simulink model "Control_Logic_e"  (R2019b)
settings: Solver=FixedStepAuto  StartTime=0  StopTime=200  FixedStep=0.1  RelTol=1e-3
values from neighbouring files (symbols this model uses):
  Sample_time = 1    [test_tool_ini.m]    (also in test_tool_initialize.m = 0.1)
undefined symbols (not defined in the file or in its folder): Aset_N1, Aset_N10, Aset_N11, Aset_N12, Aset_N2, Aset_N3, Aset_N4, Aset_N5, Aset_N6, Aset_N7, Aset_N8, Aset_N9, Dset_N1, Dset_N2
(part 1 of 3)
settings Model: Creator=M156732  LastModifiedBy=yangy
settings DataIOCC: ExternalInput=aoe_tsinghua_mhi_data  LoadExternalInput=on  ReturnWorkspaceOutputs=off
settings DebuggingCC: UnderSpecifiedDimensionMsg=warning  ArithmeticOperatorsInVariantConditions=warning
settings ModelReferenceCC: ModelReferenceNumInstancesAllowed=Single
settings SFSimCC: CustomCodeUndefinedFunction=UseInterfaceOnly

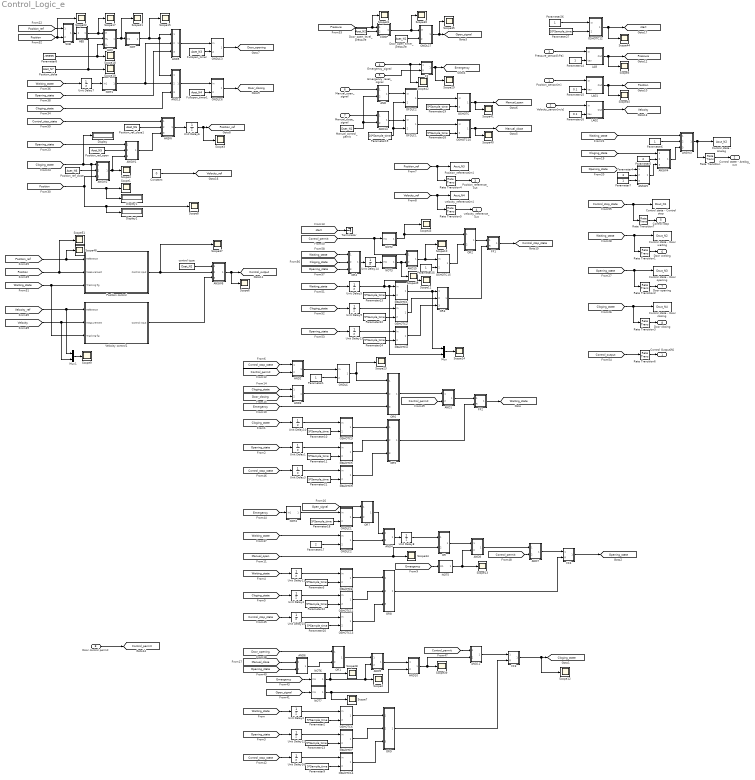
== system Control_Logic_e ==
  Position_sensor[m] : Inport  OutDataTypeStr=double  Unit=mm  PortDimensions=1  SampleTime=Sample_time
  Velocity_sensor[m/s] : Inport  Port=2  OutDataTypeStr=double  Unit=mm  PortDimensions=1  SampleTime=Sample_time
  Pressure_sensor[kPa] : Inport  Port=3  OutDataTypeStr=double  Unit=kPa  PortDimensions=1  SampleTime=Sample_time
  Emergency_signal : Inport  Port=4  OutDataTypeStr=boolean  PortDimensions=1  SampleTime=Sample_time
  Emergency_reset_signal : Inport  Port=5  OutDataTypeStr=boolean  PortDimensions=1  SampleTime=Sample_time
  Manual_open_signal : Inport  Port=6  OutDataTypeStr=boolean  PortDimensions=1  SampleTime=Sample_time
  Manual_close_signal : Inport  Port=7  OutDataTypeStr=boolean  PortDimensions=1  SampleTime=Sample_time
  Door control permit : Inport  Port=8  OutDataTypeStr=boolean  PortDimensions=1  SampleTime=Sample_time
  ABS : Subsystem
  AND : Subsystem
  AND1 : Subsystem
  AND10 : Subsystem
  AND11 : Subsystem
  AND13 : Subsystem
  AND14 : Subsystem
  AND15 : Subsystem
  AND2 : Subsystem
  AND3 : Subsystem
  AND4 : Subsystem
  AND5 : Subsystem
  AND6 : Subsystem
  AND7 : Subsystem
  AND8 : Subsystem
  AND9 : Subsystem
  ANSW : Subsystem
  ANSW1 : Subsystem
  ANSW2 : Subsystem
  ANSW3 : Subsystem
  ANSW4 : Subsystem
  ANSW5 : Subsystem
  ANSW6 : Subsystem
  COMP : Subsystem
  Constant : Constant  Value=0
  Control state - Analog : ToWorkspace  VariableName=Aout_N2  SampleTime=Sample_time
  Control state - Control stop : ToWorkspace  VariableName=Dout_N1  SampleTime=Sample_time
  Control state - Door closing : ToWorkspace  VariableName=Dout_N4  SampleTime=Sample_time
  Control state - Door opening : ToWorkspace  VariableName=Dout_N3  SampleTime=Sample_time
  Control state - Door waiting : ToWorkspace  VariableName=Dout_N2  SampleTime=Sample_time
  Display : Display
  Display1 : Display
  Display2 : Display
  Door_open_level_pressure : Constant  Value=Aset_N2  OutDataTypeStr=double  SampleTime=Sample_time
  Door_open_timer_pressure : Constant  Value=Aset_N1  OutDataTypeStr=double  SampleTime=Sample_time
  FF : Subsystem
  FF1 : Subsystem
  FF2 : Subsystem
  FF3 : Subsystem
  FF4 : Subsystem
  Fullopen_timer : Constant  Value=Aset_N3  OutDataTypeStr=double  SampleTime=Sample_time
  Fullopen_timer1 : Constant  Value=Aset_N4  OutDataTypeStr=double  SampleTime=Sample_time
  HLM : Subsystem
  LAG : Subsystem
  LAG1 : Subsystem
  LAG2 : Subsystem
  Manual_control_pemit : Constant  Value=Dset_N1  OutDataTypeStr=boolean  SampleTime=Sample_time
  Mux : Mux  Inputs=2
  Mux1 : Mux  Inputs=2
  NOT : Subsystem
  NOT1 : Subsystem
  NOT2 : Subsystem
  NOT3 : Subsystem
  NOT4 : Subsystem
  NOT5 : Subsystem
  NOT6 : Subsystem
  NOT7 : Subsystem
  OFDLC1 : Subsystem
  OFDLC2 : Subsystem
  ONDLC : Subsystem
  ONDLC1 : Subsystem
  ONDLC2 : Subsystem
  ONDLC3 : Subsystem
  ONDLC6 : Subsystem
  ONDLC7 : Subsystem
  OR : Subsystem
  OR1 : Subsystem
  OR2 : Subsystem
  OR3 : Subsystem
  OR4 : Subsystem
  OR5 : Subsystem
  OR6 : Subsystem
  OR7 : Subsystem
  OR8 : Subsystem
  OR9 : Subsystem
  OSHOTC : Subsystem
  OSHOTC1 : Subsystem
  OSHOTC10 : Subsystem
  OSHOTC11 : Subsystem
  OSHOTC12 : Subsystem
  OSHOTC13 : Subsystem
  OSHOTC14 : Subsystem
  OSHOTC15 : Subsystem
  OSHOTC2 : Subsystem
  OSHOTC3 : Subsystem
  OSHOTC4 : Subsystem
  OSHOTC5 : Subsystem
  OSHOTC6 : Subsystem
  OSHOTC7 : Subsystem
  OSHOTC8 : Subsystem
  OSHOTC9 : Subsystem
  Parameter{1,6..7,14,25} (5 alike) : Constant  OutDataTypeStr=double  SampleTime=Sample_time
  Parameter{2..3,9..13,18,20..24,28..29} (15 alike) : Constant  Value=5*Sample_time  OutDataTypeStr=double  SampleTime=Sample_time
  Parameter15 : Constant  Value=0.1  OutDataTypeStr=double  SampleTime=Sample_time
  Parameter16 : Constant  Value=0.1  OutDataTypeStr=double  SampleTime=Sample_time
  Parameter17 : Constant  Value=2  OutDataTypeStr=double  SampleTime=Sample_time
  Parameter19 : Constant  Value=10*Sample_time  OutDataTypeStr=double  SampleTime=Sample_time
  Parameter26 : Constant  OutDataTypeStr=boolean  SampleTime=Sample_time
  Parameter27 : Constant  Value=10*Sample_time  OutDataTypeStr=double  SampleTime=Sample_time
  Parameter4 : Constant  Value=3  OutDataTypeStr=double  SampleTime=Sample_time
  Parameter5 : Constant  Value=2  OutDataTypeStr=double  SampleTime=Sample_time
  Parameter8 : Constant  Value=-99999  OutDataTypeStr=double  SampleTime=Sample_time
  Position control : Subsystem
  Position_delta : Constant  Value=Aset_N7  OutDataTypeStr=double  SampleTime=Sample_time
  Position_ref_close : Constant  Value=Aset_N6  OutDataTypeStr=double  SampleTime=Sample_time
  Position_ref_close1 : Constant  Value=Aset_N6  OutDataTypeStr=double  SampleTime=Sample_time
  Position_ref_open : Constant  Value=Aset_N5  OutDataTypeStr=double  SampleTime=Sample_time
  Position_reference[m] : ToWorkspace  VariableName=Aout_N3  SampleTime=Sample_time
  Rate Transition{,1..7} (8 alike) : RateTransition  OutPortSampleTime=Sample_time
  SUB : Subsystem
  Scope{1..15,17..19,21..23,28..31,34..35,37,39..45,48..49,51} (38 alike) : Scope
  Terminator : Terminator
  Unit Delay{1..13,15..16} (15 alike) : UnitDelay  SampleTime=Sample_time  HasFrameUpgradeWarning=on
  Unit Delay14 : UnitDelay  InitialCondition=1  SampleTime=Sample_time  HasFrameUpgradeWarning=on
  Velocity control1 : Subsystem
  control type : Constant  Value=Dset_N2  OutDataTypeStr=boolean  SampleTime=Sample_time
  velocity_reference[m] : ToWorkspace  VariableName=Aout_N4  SampleTime=Sample_time
  Control Output[N] : Outport  OutDataTypeStr=double  Unit=N  SampleTime=Sample_time  VectorParamsAs1DForOutWhenUnconnected=off  LockScale=on
  Control state - Analog_out : Outport  Port=2  SampleTime=Sample_time  VectorParamsAs1DForOutWhenUnconnected=off
  Position_reference_out : Outport  Port=3  SampleTime=Sample_time  VectorParamsAs1DForOutWhenUnconnected=off
  velocity_reference_out : Outport  Port=4  SampleTime=Sample_time  VectorParamsAs1DForOutWhenUnconnected=off
  Control stop : Outport  Port=5  SampleTime=Sample_time  VectorParamsAs1DForOutWhenUnconnected=off
  Door waiting : Outport  Port=6  SampleTime=Sample_time  VectorParamsAs1DForOutWhenUnconnected=off
  Door opening : Outport  Port=7  SampleTime=Sample_time  VectorParamsAs1DForOutWhenUnconnected=off
  Door closing : Outport  Port=8  SampleTime=Sample_time  VectorParamsAs1DForOutWhenUnconnected=off
  tag scope: Cloging_state=global, Control_output=global, Control_permit=global, Control_stop_state=global, Door_closing=global, Door_opening=global, Emergency=global, Manual_close=global, Manual_open=global, Open_signal=global, Opening_state=global, Position=global, Position_ref=global, Pressure=global, Velocity=global, Velocity_ref=global, Waiting_state=global, start=global
  wires:
  FF3/1(Out1) -> [Cloging_state], Scope12/1
  FF4/1(Out1) -> [Opening_state]
  AND3/1(Out1) -> OR6/2(In2)
  [Emergency] -> OR6/3(In3)
  [Door_closing] -> AND3/2(In2)
  [Cloging_state] -> AND3/1(In1)
  [Manual_open] -> OR/2(In2), Scope34/1
  OR/1(Out) -> AND8/1(In1)
  [Door_opening] -> OR1/1(In1)
  Door_open_timer_pressure/1 -> ONDLC7/2(Tset)
  Door_open_level_pressure/1 -> COMP/2(In2)
  COMP/1(Out1) -> ONDLC7/1(In), Scope30/1
  ONDLC7/1(Out) -> Scope35/1, [Open_signal]
  FF/1(Out1) -> Scope29/1, [Emergency]
  Emergency_reset_signal/1 -> FF/2(R)
  ANSW4/1(Out1) -> ANSW3/3(InB)
  ANSW5/1(Out1) -> ANSW4/3(InB)
  Parameter4/1 -> ANSW5/2(InA)
  Parameter5/1 -> ANSW4/2(InA)
  Parameter6/1 -> ANSW3/2(InA)
  Parameter7/1 -> ANSW5/3(InB)
  ANSW3/1(Out1) -> Rate Transition/1, Control state - Analog/1
  Manual_control_pemit/1 -> AND14/2(In2), AND/2(In2)
  [Position_ref] -> SUB/1(In1)
  SUB/1(Out) -> ABS/1(In1)
  Position_delta/1 -> HLM/2(HL), Scope19/1
  Parameter8/1 -> HLM/3(LL), Scope18/1
  HLM/1(Out1) -> NOT/1(In1), Scope21/1
  Fullopen_timer/1 -> ONDLC3/2(Tset)
  [Opening_state] -> ANSW1/1(SW)
  ANSW2/1(Out1) -> ANSW1/3(InB), Scope4/1
  [Cloging_state] -> Display/1, Display1/1, Scope1/1, ANSW2/1(SW)
  Position_ref_open/1 -> ANSW1/2(InA)
  Position_ref_close/1 -> ANSW2/2(InA)
  [Position] -> ANSW2/3(InB), Display2/1, Scope8/1
  Fullopen_timer1/1 -> ONDLC6/2(Tset)
  [Waiting_state] -> Rate Transition1/1, Control state - Door waiting/1
  [Opening_state] -> Rate Transition2/1, Control state - Door opening/1
  [Cloging_state] -> Rate Transition3/1, Control state - Door closing/1
  [Position] -> SUB/2(In2), Scope22/1
  [Pressure] -> COMP/1(In1), Scope31/1
  AND2/1(Out1) -> ONDLC/1(In)
  ONDLC/1(Out) -> OR6/1(In1), Scope23/1
  ABS/1(Out1) -> HLM/1(In), Scope17/1
  ONDLC3/1(Out) -> [Door_opening]
  ONDLC6/1(Out) -> [Door_closing]
  [Waiting_state] -> Unit Delay7/1
  NOT/1(Out1) -> Scope15/1, AND13/1(In1), AND5/1(In1)
  AND5/1(Out1) -> ONDLC3/1(In)
  NOT1/1(Out1) -> AND5/2(In2), AND13/2(In2)
  Unit Delay7/1 -> NOT1/1(In1)
  AND4/1(Out1) -> Unit Delay8/1
  Unit Delay8/1 -> OR/1(In1)
  [Opening_state] -> AND5/3(In3)
  [Cloging_state] -> AND13/3(In3)
  AND13/1(Out1) -> ONDLC6/1(In)
  [Opening_state] -> Unit Delay1/1
  [Cloging_state] -> Unit Delay10/1
  Unit Delay10/1 -> OSHOTC3/1(In)
  Unit Delay1/1 -> OSHOTC5/1(In)
  OSHOTC5/1(Out) -> OR5/2(In2)
  OSHOTC11/1(Out) -> OR8/2(In2)
  [Waiting_state] -> Unit Delay11/1
  OSHOTC8/1(Out) -> OR8/1(In1)
  Unit Delay11/1 -> OSHOTC8/1(In)
  [Cloging_state] -> Unit Delay4/1
  Unit Delay4/1 -> OSHOTC11/1(In)
  [Waiting_state] -> Unit Delay2/1
  Parameter2/1 -> OSHOTC6/2(Tset)
  OSHOTC6/1(Out) -> OR9/1(In1)
  Parameter13/1 -> OSHOTC7/2(Tset)
  [Opening_state] -> Unit Delay12/1
  OSHOTC7/1(Out) -> OR9/2(In2)
  Unit Delay2/1 -> OSHOTC6/1(In)
  Unit Delay12/1 -> OSHOTC7/1(In)
  Pressure_sensor[kPa]/1 -> LAG/1(In)
  LAG/1(Out) -> [Pressure], Scope5/1
  LAG1/1(Out) -> Scope45/1, [Position]
  Position_sensor[m]/1 -> LAG1/1(In)
  LAG2/1(Out) -> [Velocity]
  Velocity_sensor[m/s]/1 -> LAG2/1(In)
  Parameter14/1 -> LAG/2(tau)
  Parameter15/1 -> LAG1/2(tau)
  Parameter16/1 -> LAG2/2(tau)
  [Waiting_state] -> ANSW3/1(SW)
  [Cloging_state] -> ANSW4/1(SW)
  [Opening_state] -> ANSW5/1(SW)
  Rate Transition/1 -> Control state - Analog_out/1
  Rate Transition1/1 -> Door waiting/1
  Rate Transition2/1 -> Door opening/1
  Rate Transition3/1 -> Door closing/1
  [Waiting_state] -> ONDLC2/1(In)
  ONDLC2/1(Out) -> AND4/2(In2)
  [Position_ref] -> Rate Transition4/1, Position_reference[m]/1
  Rate Transition4/1 -> Position_reference_out/1
  Rate Transition5/1 -> velocity_reference_out/1
  [Velocity_ref] -> velocity_reference[m]/1, Rate Transition5/1
  [Emergency] -> NOT5/1(In1)
  NOT5/1(Out1) -> AND8/2(In2), Scope13/1
  [Emergency] -> NOT6/1(In1)
  OR1/1(Out) -> AND9/1(In1)
  OR7/1(Out) -> AND4/1(In1)
  [Open_signal] -> OR7/1(In1)
  [Emergency] -> NOT4/1(In1)
  Parameter18/1 -> ONDLC1/2(Tset)
  ONDLC1/1(Out) -> OR7/2(In2)
  NOT4/1(Out1) -> ONDLC1/1(In)
  Manual_open_signal/1 -> AND/1(In1)
  Manual_close_signal/1 -> AND14/1(In1)
  AND14/1(Out1) -> OFDLC1/1(In)
  AND/1(Out1) -> OFDLC2/1(In)
  Parameter19/1 -> OFDLC1/2(Tset), OFDLC2/2(Tset)
  AND6/1(Out1) -> OR1/2(In2)
  [Opening_state] -> AND6/2(In2)
  [Open_signal] -> NOT7/1(In1)
  NOT7/1(Out1) -> AND10/2(In2), Scope7/1
  NOT6/1(Out1) -> Scope28/1, AND9/2(In2), Scope2/1
  Emergency_signal/1 -> FF/1(SS), Scope42/1
  AND9/1(Out1) -> AND10/1(In1)
  Door control permit/1 -> [Control_permit]
  OSHOTC13/1(Out) -> OR8/3(In3)
  OSHOTC9/1(Out) -> OR5/3(In3)
  AND11/1(Out1) -> FF3/1(SS)
  AND10/1(Out1) -> AND11/2(In2), Scope39/1
  [Control_permit] -> AND11/1(In1)
  AND8/1(Out1) -> AND7/1(In1)
  [Control_permit] -> AND7/2(In2)
  [Control_permit] -> AND1/2(In2)
  OR6/1(Out) -> AND1/1(In1)
  AND1/1(Out1) -> FF2/1(SS)
  FF1/1(Out1) -> [Control_stop_state]
  [Control_permit] -> AND15/1(In1), NOT2/1(In1)
  OSHOTC4/1(Out) -> OR3/3(In3)
  Unit Delay9/1 -> OSHOTC2/1(In)
  [Cloging_state] -> Unit Delay9/1
  Unit Delay5/1 -> Scope11/1, Mux/2, OSHOTC1/1(In)
  OSHOTC1/1(Out) -> Mux/1, OR3/1(In1)
  [Waiting_state] -> Unit Delay5/1
  OSHOTC2/1(Out) -> OR3/2(In2)
  Unit Delay13/1 -> OSHOTC4/1(In)
  [Opening_state] -> Unit Delay13/1
  OR3/1(Out) -> FF1/2(R)
  Rate Transition6/1 -> Control Output[N]/1
  [Control_output] -> Rate Transition6/1
  Rate Transition7/1 -> Control stop/1
  [Control_stop_state] -> Control state - Control stop/1, Rate Transition7/1
  Constant/1 -> [Velocity_ref]
  NOT2/1(Out1) -> OR2/1(In1), Scope43/1
  OR2/1(Out) -> FF1/1(SS)
  [Cloging_state] -> OR4/2(In2)
  Unit Delay14/1 -> NOT3/1(In1)
  [Waiting_state] -> OR4/1(In1)
  OR4/1(Out) -> Unit Delay14/1
  [Opening_state] -> OR4/3(In3)
  [Control_stop_state] -> AND2/1(In1)
  [Control_permit] -> AND2/2(In2)
  Parameter26/1 -> OSHOTC12/1(In)
  OSHOTC12/1(Out) -> Scope44/1, [start]
  AND15/1(Out1) -> Scope10/1, OSHOTC15/1(In)
  NOT3/1(Out1) -> AND15/2(In2), Scope49/1
  Parameter21/1 -> OSHOTC9/2(Tset)
  Unit Delay3/1 -> OSHOTC9/1(In)
  [Control_stop_state] -> Unit Delay3/1
  [Control_stop_state] -> Unit Delay15/1
  Unit Delay15/1 -> OSHOTC13/1(In)
  Parameter20/1 -> OSHOTC13/2(Tset)
  Unit Delay16/1 -> OSHOTC14/1(In)
  [Control_stop_state] -> Unit Delay16/1
  ANSW1/1(Out1) -> ANSW/3(InB)
  [Control_stop_state] -> ANSW/1(SW)
  Position_ref_close1/1 -> ANSW/2(InA)
  [Manual_close] -> AND6/1(In1)
  Parameter28/1 -> OSHOTC10/2(Tset)
  OFDLC1/1(Out) -> OSHOTC10/1(In)
  OFDLC2/1(Out) -> OSHOTC/1(In)
  Parameter29/1 -> OSHOTC/2(Tset)
  OSHOTC/1(Out) -> [Manual_open], Scope41/1
  OSHOTC10/1(Out) -> Scope40/1, [Manual_close]
  [start] -> Terminator/1
  ANSW/1(Out1) -> Unit Delay6/1
  Unit Delay6/1 -> Scope3/1, [Position_ref]
  Parameter27/1 -> OSHOTC12/2(Tset)
  Parameter23/1 -> OSHOTC1/2(Tset)
  Parameter22/1 -> OSHOTC2/2(Tset)
  Parameter24/1 -> OSHOTC4/2(Tset)
  OSHOTC3/1(Out) -> OR5/1(In1)
  Parameter10/1 -> OSHOTC3/2(Tset)
  Parameter11/1 -> OSHOTC5/2(Tset)
  Parameter3/1 -> OSHOTC8/2(Tset)
  Parameter12/1 -> OSHOTC11/2(Tset)
  OSHOTC14/1(Out) -> OR9/3(In3)
  Parameter9/1 -> OSHOTC14/2(Tset)
  AND7/1(Out1) -> FF4/1(SS)
  OR5/1(Out) -> FF2/2(R)
  OR8/1(Out) -> FF4/2(R)
  OR9/1(Out) -> FF3/2(R)
  OSHOTC15/1(Out) -> OR2/2(In2)
  FF2/1(Out1) -> [Waiting_state]
  control type/1 -> ANSW6/1(SW)
  [Velocity] -> Velocity control1/2(Measurement), Mux1/2
  Mux1/1 -> Scope9/1
  ANSW6/1(Out1) -> [Control_output], Scope6/1
  [Velocity_ref] -> Velocity control1/1(Reference), Mux1/1
  [Position] -> Scope51/1, Position control/2(Measurement)
  Position control/1(Control input) -> ANSW6/2(InA), Scope37/1
  [Position_ref] -> Scope48/1, Position control/1(Reference)
  [Waiting_state] -> Velocity control1/3(Tracking flg), Position control/3(Tracking flg)
  Velocity control1/1(Control input) -> ANSW6/3(InB)
  Mux/1 -> Scope14/1
  Parameter25/1 -> OSHOTC15/2(Tset)
  Parameter1/1 -> ONDLC/2(Tset)
  Parameter17/1 -> ONDLC2/2(Tset)

== system Control_Logic_e/ABS ==
  In1 : Inport
  ABS : MATLAB Function  TreatAsAtomicUnit=on
  Out1 : Outport  VectorParamsAs1DForOutWhenUnconnected=off
  wires:
  ABS/1(y) -> Out1/1
  In1/1 -> ABS/1(u)

== system Control_Logic_e/AND ==
  In1 : Inport
  In2 : Inport  Port=2
  AND : MATLAB Function  TreatAsAtomicUnit=on
  Cast To Boolean : DataTypeConversion  OutDataTypeStr=boolean
  Cast To Double : DataTypeConversion  OutDataTypeStr=double
  Cast To Double1 : DataTypeConversion  OutDataTypeStr=double
  Mux : Mux  Inputs=2
  Out1 : Outport  VectorParamsAs1DForOutWhenUnconnected=off
  wires:
  In2/1 -> Cast To Double1/1
  In1/1 -> Cast To Double/1
  Mux/1 -> AND/1(u)
  AND/1(y) -> Cast To Boolean/1
  Cast To Boolean/1 -> Out1/1
  Cast To Double/1 -> Mux/1
  Cast To Double1/1 -> Mux/2

== system Control_Logic_e/AND1 ==
  In1 : Inport
  In2 : Inport  Port=2
  AND : MATLAB Function  TreatAsAtomicUnit=on
  Cast To Boolean : DataTypeConversion  OutDataTypeStr=boolean
  Cast To Double : DataTypeConversion  OutDataTypeStr=double
  Cast To Double1 : DataTypeConversion  OutDataTypeStr=double
  Mux : Mux  Inputs=2
  Out1 : Outport  VectorParamsAs1DForOutWhenUnconnected=off
  wires:
  In2/1 -> Cast To Double1/1
  In1/1 -> Cast To Double/1
  Mux/1 -> AND/1(u)
  AND/1(y) -> Cast To Boolean/1
  Cast To Boolean/1 -> Out1/1
  Cast To Double/1 -> Mux/1
  Cast To Double1/1 -> Mux/2

== system Control_Logic_e/AND10 ==
  In1 : Inport
  In2 : Inport  Port=2
  AND : MATLAB Function  TreatAsAtomicUnit=on
  Cast To Boolean : DataTypeConversion  OutDataTypeStr=boolean
  Cast To Double : DataTypeConversion  OutDataTypeStr=double
  Cast To Double1 : DataTypeConversion  OutDataTypeStr=double
  Mux : Mux  Inputs=2
  Out1 : Outport  VectorParamsAs1DForOutWhenUnconnected=off
  wires:
  Cast To Double1/1 -> Mux/2
  Cast To Double/1 -> Mux/1
  Cast To Boolean/1 -> Out1/1
  AND/1(y) -> Cast To Boolean/1
  Mux/1 -> AND/1(u)
  In1/1 -> Cast To Double/1
  In2/1 -> Cast To Double1/1

== system Control_Logic_e/AND11 ==
  In1 : Inport
  In2 : Inport  Port=2
  AND : MATLAB Function  TreatAsAtomicUnit=on
  Cast To Boolean : DataTypeConversion  OutDataTypeStr=boolean
  Cast To Double : DataTypeConversion  OutDataTypeStr=double
  Cast To Double1 : DataTypeConversion  OutDataTypeStr=double
  Mux : Mux  Inputs=2
  Out1 : Outport  VectorParamsAs1DForOutWhenUnconnected=off
  wires:
  Cast To Double1/1 -> Mux/2
  Cast To Double/1 -> Mux/1
  Cast To Boolean/1 -> Out1/1
  AND/1(y) -> Cast To Boolean/1
  Mux/1 -> AND/1(u)
  In1/1 -> Cast To Double/1
  In2/1 -> Cast To Double1/1

== system Control_Logic_e/AND13 ==
  In1 : Inport
  In2 : Inport  Port=2
  In3 : Inport  Port=3
  AND : MATLAB Function  TreatAsAtomicUnit=on
  Cast To Boolean : DataTypeConversion  OutDataTypeStr=boolean
  Cast To Double : DataTypeConversion  OutDataTypeStr=double
  Cast To Double1 : DataTypeConversion  OutDataTypeStr=double
  Cast To Double2 : DataTypeConversion  OutDataTypeStr=double
  Mux : Mux  Inputs=3
  Out1 : Outport  VectorParamsAs1DForOutWhenUnconnected=off
  wires:
  In3/1 -> Cast To Double2/1
  Cast To Double1/1 -> Mux/2
  Cast To Double/1 -> Mux/1
  Mux/1 -> AND/1(u)
  Cast To Boolean/1 -> Out1/1
  AND/1(y) -> Cast To Boolean/1
  In1/1 -> Cast To Double/1
  In2/1 -> Cast To Double1/1
  Cast To Double2/1 -> Mux/3

== system Control_Logic_e/AND14 ==
  In1 : Inport
  In2 : Inport  Port=2
  AND : MATLAB Function  TreatAsAtomicUnit=on
  Cast To Boolean : DataTypeConversion  OutDataTypeStr=boolean
  Cast To Double : DataTypeConversion  OutDataTypeStr=double
  Cast To Double1 : DataTypeConversion  OutDataTypeStr=double
  Mux : Mux  Inputs=2
  Out1 : Outport  VectorParamsAs1DForOutWhenUnconnected=off
  wires:
  In2/1 -> Cast To Double1/1
  In1/1 -> Cast To Double/1
  Mux/1 -> AND/1(u)
  AND/1(y) -> Cast To Boolean/1
  Cast To Boolean/1 -> Out1/1
  Cast To Double/1 -> Mux/1
  Cast To Double1/1 -> Mux/2

== system Control_Logic_e/AND15 ==
  In1 : Inport
  In2 : Inport  Port=2
  AND : MATLAB Function  TreatAsAtomicUnit=on
  Cast To Boolean : DataTypeConversion  OutDataTypeStr=boolean
  Cast To Double : DataTypeConversion  OutDataTypeStr=double
  Cast To Double1 : DataTypeConversion  OutDataTypeStr=double
  Mux : Mux  Inputs=2
  Out1 : Outport  VectorParamsAs1DForOutWhenUnconnected=off
  wires:
  In2/1 -> Cast To Double1/1
  In1/1 -> Cast To Double/1
  Mux/1 -> AND/1(u)
  AND/1(y) -> Cast To Boolean/1
  Cast To Boolean/1 -> Out1/1
  Cast To Double/1 -> Mux/1
  Cast To Double1/1 -> Mux/2

== system Control_Logic_e/AND2 ==
  In1 : Inport
  In2 : Inport  Port=2
  AND : MATLAB Function  TreatAsAtomicUnit=on
  Cast To Boolean : DataTypeConversion  OutDataTypeStr=boolean
  Cast To Double : DataTypeConversion  OutDataTypeStr=double
  Cast To Double1 : DataTypeConversion  OutDataTypeStr=double
  Mux : Mux  Inputs=2
  Out1 : Outport  VectorParamsAs1DForOutWhenUnconnected=off
  wires:
  In2/1 -> Cast To Double1/1
  In1/1 -> Cast To Double/1
  Mux/1 -> AND/1(u)
  AND/1(y) -> Cast To Boolean/1
  Cast To Boolean/1 -> Out1/1
  Cast To Double/1 -> Mux/1
  Cast To Double1/1 -> Mux/2

== system Control_Logic_e/AND3 ==
  In1 : Inport
  In2 : Inport  Port=2
  AND : MATLAB Function  TreatAsAtomicUnit=on
  Cast To Boolean : DataTypeConversion  OutDataTypeStr=boolean
  Cast To Double : DataTypeConversion  OutDataTypeStr=double
  Cast To Double1 : DataTypeConversion  OutDataTypeStr=double
  Mux : Mux  Inputs=2
  Out1 : Outport  VectorParamsAs1DForOutWhenUnconnected=off
  wires:
  In2/1 -> Cast To Double1/1
  In1/1 -> Cast To Double/1
  Mux/1 -> AND/1(u)
  AND/1(y) -> Cast To Boolean/1
  Cast To Boolean/1 -> Out1/1
  Cast To Double/1 -> Mux/1
  Cast To Double1/1 -> Mux/2

== system Control_Logic_e/AND4 ==
  In1 : Inport
  In2 : Inport  Port=2
  AND : MATLAB Function  TreatAsAtomicUnit=on
  Cast To Boolean : DataTypeConversion  OutDataTypeStr=boolean
  Cast To Double : DataTypeConversion  OutDataTypeStr=double
  Cast To Double1 : DataTypeConversion  OutDataTypeStr=double
  Mux : Mux  Inputs=2
  Out1 : Outport  VectorParamsAs1DForOutWhenUnconnected=off
  wires:
  In2/1 -> Cast To Double1/1
  In1/1 -> Cast To Double/1
  Mux/1 -> AND/1(u)
  AND/1(y) -> Cast To Boolean/1
  Cast To Boolean/1 -> Out1/1
  Cast To Double/1 -> Mux/1
  Cast To Double1/1 -> Mux/2

== system Control_Logic_e/AND5 ==
  In1 : Inport
  In2 : Inport  Port=2
  In3 : Inport  Port=3
  AND : MATLAB Function  TreatAsAtomicUnit=on
  Cast To Boolean : DataTypeConversion  OutDataTypeStr=boolean
  Cast To Double : DataTypeConversion  OutDataTypeStr=double
  Cast To Double1 : DataTypeConversion  OutDataTypeStr=double
  Cast To Double2 : DataTypeConversion  OutDataTypeStr=double
  Mux : Mux  Inputs=3
  Out1 : Outport  VectorParamsAs1DForOutWhenUnconnected=off
  wires:
  In2/1 -> Cast To Double1/1
  In1/1 -> Cast To Double/1
  AND/1(y) -> Cast To Boolean/1
  Cast To Boolean/1 -> Out1/1
  Mux/1 -> AND/1(u)
  Cast To Double/1 -> Mux/1
  Cast To Double1/1 -> Mux/2
  In3/1 -> Cast To Double2/1
  Cast To Double2/1 -> Mux/3

== system Control_Logic_e/AND6 ==
  In1 : Inport
  In2 : Inport  Port=2
  AND : MATLAB Function  TreatAsAtomicUnit=on
  Cast To Boolean : DataTypeConversion  OutDataTypeStr=boolean
  Cast To Double : DataTypeConversion  OutDataTypeStr=double
  Cast To Double1 : DataTypeConversion  OutDataTypeStr=double
  Mux : Mux  Inputs=2
  Out1 : Outport  VectorParamsAs1DForOutWhenUnconnected=off
  wires:
  Cast To Double1/1 -> Mux/2
  Cast To Double/1 -> Mux/1
  Cast To Boolean/1 -> Out1/1
  AND/1(y) -> Cast To Boolean/1
  Mux/1 -> AND/1(u)
  In1/1 -> Cast To Double/1
  In2/1 -> Cast To Double1/1

== system Control_Logic_e/AND7 ==
  In1 : Inport
  In2 : Inport  Port=2
  AND : MATLAB Function  TreatAsAtomicUnit=on
  Cast To Boolean : DataTypeConversion  OutDataTypeStr=boolean
  Cast To Double : DataTypeConversion  OutDataTypeStr=double
  Cast To Double1 : DataTypeConversion  OutDataTypeStr=double
  Mux : Mux  Inputs=2
  Out1 : Outport  VectorParamsAs1DForOutWhenUnconnected=off
  wires:
  In2/1 -> Cast To Double1/1
  In1/1 -> Cast To Double/1
  Mux/1 -> AND/1(u)
  AND/1(y) -> Cast To Boolean/1
  Cast To Boolean/1 -> Out1/1
  Cast To Double/1 -> Mux/1
  Cast To Double1/1 -> Mux/2

== system Control_Logic_e/AND8 ==
  In1 : Inport
  In2 : Inport  Port=2
  AND : MATLAB Function  TreatAsAtomicUnit=on
  Cast To Boolean : DataTypeConversion  OutDataTypeStr=boolean
  Cast To Double : DataTypeConversion  OutDataTypeStr=double
  Cast To Double1 : DataTypeConversion  OutDataTypeStr=double
  Mux : Mux  Inputs=2
  Out1 : Outport  VectorParamsAs1DForOutWhenUnconnected=off
  wires:
  In2/1 -> Cast To Double1/1
  In1/1 -> Cast To Double/1
  Mux/1 -> AND/1(u)
  AND/1(y) -> Cast To Boolean/1
  Cast To Boolean/1 -> Out1/1
  Cast To Double/1 -> Mux/1
  Cast To Double1/1 -> Mux/2

== system Control_Logic_e/AND9 ==
  In1 : Inport
  In2 : Inport  Port=2
  AND : MATLAB Function  TreatAsAtomicUnit=on
  Cast To Boolean : DataTypeConversion  OutDataTypeStr=boolean
  Cast To Double : DataTypeConversion  OutDataTypeStr=double
  Cast To Double1 : DataTypeConversion  OutDataTypeStr=double
  Mux : Mux  Inputs=2
  Out1 : Outport  VectorParamsAs1DForOutWhenUnconnected=off
  wires:
  Cast To Double1/1 -> Mux/2
  Cast To Double/1 -> Mux/1
  Cast To Boolean/1 -> Out1/1
  AND/1(y) -> Cast To Boolean/1
  Mux/1 -> AND/1(u)
  In1/1 -> Cast To Double/1
  In2/1 -> Cast To Double1/1

== system Control_Logic_e/ANSW ==
  SW : Inport
  InA : Inport  Port=2
  InB : Inport  Port=3
  Cast To Double : DataTypeConversion  OutDataTypeStr=double
  MATLAB Function : MATLAB Function  TreatAsAtomicUnit=on
  Mux : Mux  Inputs=3
  Out1 : Outport  VectorParamsAs1DForOutWhenUnconnected=off
  wires:
  Cast To Double/1 -> Mux/1
  Mux/1 -> MATLAB Function/1(u)
  InB/1 -> Mux/3
  InA/1 -> Mux/2
  MATLAB Function/1(y) -> Out1/1
  SW/1 -> Cast To Double/1

== system Control_Logic_e/ANSW1 ==
  SW : Inport
  InA : Inport  Port=2
  InB : Inport  Port=3
  Cast To Double : DataTypeConversion  OutDataTypeStr=double
  MATLAB Function : MATLAB Function  TreatAsAtomicUnit=on
  Mux : Mux  Inputs=3
  Out1 : Outport  VectorParamsAs1DForOutWhenUnconnected=off
  wires:
  Cast To Double/1 -> Mux/1
  Mux/1 -> MATLAB Function/1(u)
  InB/1 -> Mux/3
  InA/1 -> Mux/2
  MATLAB Function/1(y) -> Out1/1
  SW/1 -> Cast To Double/1

== system Control_Logic_e/ANSW2 ==
  SW : Inport
  InA : Inport  Port=2
  InB : Inport  Port=3
  Cast To Double : DataTypeConversion  OutDataTypeStr=double
  MATLAB Function : MATLAB Function  TreatAsAtomicUnit=on
  Mux : Mux  Inputs=3
  Out1 : Outport  VectorParamsAs1DForOutWhenUnconnected=off
  wires:
  Cast To Double/1 -> Mux/1
  Mux/1 -> MATLAB Function/1(u)
  InB/1 -> Mux/3
  InA/1 -> Mux/2
  MATLAB Function/1(y) -> Out1/1
  SW/1 -> Cast To Double/1

== system Control_Logic_e/ANSW3 ==
  SW : Inport
  InA : Inport  Port=2
  InB : Inport  Port=3
  Cast To Double : DataTypeConversion  OutDataTypeStr=double
  MATLAB Function : MATLAB Function  TreatAsAtomicUnit=on
  Mux : Mux  Inputs=3
  Out1 : Outport  VectorParamsAs1DForOutWhenUnconnected=off
  wires:
  Cast To Double/1 -> Mux/1
  Mux/1 -> MATLAB Function/1(u)
  InB/1 -> Mux/3
  InA/1 -> Mux/2
  MATLAB Function/1(y) -> Out1/1
  SW/1 -> Cast To Double/1

== system Control_Logic_e/ANSW4 ==
  SW : Inport
  InA : Inport  Port=2
  InB : Inport  Port=3
  Cast To Double : DataTypeConversion  OutDataTypeStr=double
  MATLAB Function : MATLAB Function  TreatAsAtomicUnit=on
  Mux : Mux  Inputs=3
  Out1 : Outport  VectorParamsAs1DForOutWhenUnconnected=off
  wires:
  Cast To Double/1 -> Mux/1
  Mux/1 -> MATLAB Function/1(u)
  InB/1 -> Mux/3
  InA/1 -> Mux/2
  MATLAB Function/1(y) -> Out1/1
  SW/1 -> Cast To Double/1

== system Control_Logic_e/ANSW5 ==
  SW : Inport
  InA : Inport  Port=2
  InB : Inport  Port=3
  Cast To Double : DataTypeConversion  OutDataTypeStr=double
  MATLAB Function : MATLAB Function  TreatAsAtomicUnit=on
  Mux : Mux  Inputs=3
  Out1 : Outport  VectorParamsAs1DForOutWhenUnconnected=off
  wires:
  Cast To Double/1 -> Mux/1
  Mux/1 -> MATLAB Function/1(u)
  InB/1 -> Mux/3
  InA/1 -> Mux/2
  MATLAB Function/1(y) -> Out1/1
  SW/1 -> Cast To Double/1

== system Control_Logic_e/ANSW6 ==
  SW : Inport
  InA : Inport  Port=2
  InB : Inport  Port=3
  Cast To Double : DataTypeConversion  OutDataTypeStr=double
  MATLAB Function : MATLAB Function  TreatAsAtomicUnit=on
  Mux : Mux  Inputs=3
  Out1 : Outport  VectorParamsAs1DForOutWhenUnconnected=off
  wires:
  Cast To Double/1 -> Mux/1
  Mux/1 -> MATLAB Function/1(u)
  InB/1 -> Mux/3
  InA/1 -> Mux/2
  MATLAB Function/1(y) -> Out1/1
  SW/1 -> Cast To Double/1

== system Control_Logic_e/COMP ==
  In1 : Inport
  In2 : Inport  Port=2
  COMP : MATLAB Function  TreatAsAtomicUnit=on
  Cast To Boolean : DataTypeConversion  OutDataTypeStr=boolean
  Mux : Mux  Inputs=2
  Out1 : Outport  VectorParamsAs1DForOutWhenUnconnected=off
  wires:
  In2/1 -> Mux/2
  Cast To Boolean/1 -> Out1/1
  In1/1 -> Mux/1
  Mux/1 -> COMP/1(u)
  COMP/1(y) -> Cast To Boolean/1

== system Control_Logic_e/FF ==
  SS : Inport
  R : Inport  Port=2
  Cast To Boolean : DataTypeConversion  OutDataTypeStr=boolean
  Cast To Double : DataTypeConversion  OutDataTypeStr=double
  FF : MATLAB Function  TreatAsAtomicUnit=on
  Memory : Memory  InheritSampleTime=on
  Mux : Mux  Inputs=2
  Out1 : Outport  VectorParamsAs1DForOutWhenUnconnected=off
  wires:
  FF/1(y) -> Memory/1, Cast To Boolean/1
  SS/1 -> Mux/1
  R/1 -> Mux/2
  Mux/1 -> Cast To Double/1
  Cast To Boolean/1 -> Out1/1
  Cast To Double/1 -> FF/1(u)
  Memory/1 -> FF/2(old)

== system Control_Logic_e/FF1 ==
  SS : Inport
  R : Inport  Port=2
  Cast To Boolean : DataTypeConversion  OutDataTypeStr=boolean
  Cast To Double : DataTypeConversion  OutDataTypeStr=double
  FF : MATLAB Function  TreatAsAtomicUnit=on
  Memory : Memory  InheritSampleTime=on
  Mux : Mux  Inputs=2
  Out1 : Outport  VectorParamsAs1DForOutWhenUnconnected=off
  wires:
  FF/1(y) -> Memory/1, Cast To Boolean/1
  SS/1 -> Mux/1
  R/1 -> Mux/2
  Mux/1 -> Cast To Double/1
  Cast To Boolean/1 -> Out1/1
  Cast To Double/1 -> FF/1(u)
  Memory/1 -> FF/2(old)

== system Control_Logic_e/FF2 ==
  SS : Inport
  R : Inport  Port=2
  Cast To Boolean : DataTypeConversion  OutDataTypeStr=boolean
  Cast To Double : DataTypeConversion  OutDataTypeStr=double
  FF : MATLAB Function  TreatAsAtomicUnit=on
  Memory : Memory  InheritSampleTime=on
  Mux : Mux  Inputs=2
  Out1 : Outport  VectorParamsAs1DForOutWhenUnconnected=off
  wires:
  FF/1(y) -> Memory/1, Cast To Boolean/1
  SS/1 -> Mux/1
  R/1 -> Mux/2
  Mux/1 -> Cast To Double/1
  Cast To Boolean/1 -> Out1/1
  Cast To Double/1 -> FF/1(u)
  Memory/1 -> FF/2(old)

== system Control_Logic_e/FF3 ==
  SS : Inport
  R : Inport  Port=2
  Cast To Boolean : DataTypeConversion  OutDataTypeStr=boolean
  Cast To Double : DataTypeConversion  OutDataTypeStr=double
  FF : MATLAB Function  TreatAsAtomicUnit=on
  Memory : Memory  InheritSampleTime=on
  Mux : Mux  Inputs=2
  Out1 : Outport  VectorParamsAs1DForOutWhenUnconnected=off
  wires:
  FF/1(y) -> Memory/1, Cast To Boolean/1
  SS/1 -> Mux/1
  R/1 -> Mux/2
  Mux/1 -> Cast To Double/1
  Cast To Boolean/1 -> Out1/1
  Cast To Double/1 -> FF/1(u)
  Memory/1 -> FF/2(old)

== system Control_Logic_e/FF4 ==
  SS : Inport
  R : Inport  Port=2
  Cast To Boolean : DataTypeConversion  OutDataTypeStr=boolean
  Cast To Double : DataTypeConversion  OutDataTypeStr=double
  FF : MATLAB Function  TreatAsAtomicUnit=on
  Memory : Memory  InheritSampleTime=on
  Mux : Mux  Inputs=2
  Out1 : Outport  VectorParamsAs1DForOutWhenUnconnected=off
  wires:
  FF/1(y) -> Memory/1, Cast To Boolean/1
  SS/1 -> Mux/1
  R/1 -> Mux/2
  Mux/1 -> Cast To Double/1
  Cast To Boolean/1 -> Out1/1
  Cast To Double/1 -> FF/1(u)
  Memory/1 -> FF/2(old)

== system Control_Logic_e/HLM ==
  In : Inport
  HL : Inport  Port=2
  LL : Inport  Port=3
  Cast To Boolean : DataTypeConversion  OutDataTypeStr=boolean
  HLM : MATLAB Function  TreatAsAtomicUnit=on
  Mux : Mux  Inputs=3
  Out1 : Outport  VectorParamsAs1DForOutWhenUnconnected=off
  wires:
  HLM/1(y) -> Cast To Boolean/1
  Mux/1 -> HLM/1(u)
  Cast To Boolean/1 -> Out1/1
  In/1 -> Mux/1
  HL/1 -> Mux/2
  LL/1 -> Mux/3

== system Control_Logic_e/LAG ==
  In : Inport
  tau : Inport  Port=2
  LAG : MATLAB Function  TreatAsAtomicUnit=on
  Memory4 : Memory  InheritSampleTime=on
  Mux3 : Mux  Inputs=3
  dt2 : Constant  Value=Sample_time  OutDataTypeStr=double  SampleTime=Sample_time
  Out : Outport  VectorParamsAs1DForOutWhenUnconnected=off
  wires:
  Mux3/1 -> LAG/1(u)
  In/1 -> Mux3/1
  tau/1 -> Mux3/2
  LAG/1(y) -> Out/1, Memory4/1
  Memory4/1 -> LAG/2(old)
  dt2/1 -> Mux3/3

== system Control_Logic_e/LAG1 ==
  In : Inport
  tau : Inport  Port=2
  LAG : MATLAB Function  TreatAsAtomicUnit=on
  Memory4 : Memory  InheritSampleTime=on
  Mux3 : Mux  Inputs=3
  dt2 : Constant  Value=Sample_time  OutDataTypeStr=double  SampleTime=Sample_time
  Out : Outport  VectorParamsAs1DForOutWhenUnconnected=off
  wires:
  Mux3/1 -> LAG/1(u)
  In/1 -> Mux3/1
  tau/1 -> Mux3/2
  LAG/1(y) -> Out/1, Memory4/1
  Memory4/1 -> LAG/2(old)
  dt2/1 -> Mux3/3

== system Control_Logic_e/LAG2 ==
  In : Inport
  tau : Inport  Port=2
  LAG : MATLAB Function  TreatAsAtomicUnit=on
  Memory4 : Memory  InheritSampleTime=on
  Mux3 : Mux  Inputs=3
  dt2 : Constant  Value=Sample_time  OutDataTypeStr=double  SampleTime=Sample_time
  Out : Outport  VectorParamsAs1DForOutWhenUnconnected=off
  wires:
  Mux3/1 -> LAG/1(u)
  In/1 -> Mux3/1
  tau/1 -> Mux3/2
  LAG/1(y) -> Out/1, Memory4/1
  Memory4/1 -> LAG/2(old)
  dt2/1 -> Mux3/3

== system Control_Logic_e/NOT ==
  In1 : Inport
  Cast To Boolean : DataTypeConversion  OutDataTypeStr=boolean
  Cast To Double : DataTypeConversion  OutDataTypeStr=double
  NOT : MATLAB Function  TreatAsAtomicUnit=on
  Out1 : Outport  VectorParamsAs1DForOutWhenUnconnected=off
  wires:
  In1/1 -> Cast To Double/1
  NOT/1(y) -> Cast To Boolean/1
  Cast To Boolean/1 -> Out1/1
  Cast To Double/1 -> NOT/1(u)

== system Control_Logic_e/NOT1 ==
  In1 : Inport
  Cast To Boolean : DataTypeConversion  OutDataTypeStr=boolean
  Cast To Double : DataTypeConversion  OutDataTypeStr=double
  NOT : MATLAB Function  TreatAsAtomicUnit=on
  Out1 : Outport  VectorParamsAs1DForOutWhenUnconnected=off
  wires:
  In1/1 -> Cast To Double/1
  NOT/1(y) -> Cast To Boolean/1
  Cast To Boolean/1 -> Out1/1
  Cast To Double/1 -> NOT/1(u)

== system Control_Logic_e/NOT2 ==
  In1 : Inport
  Cast To Boolean : DataTypeConversion  OutDataTypeStr=boolean
  Cast To Double : DataTypeConversion  OutDataTypeStr=double
  NOT : MATLAB Function  TreatAsAtomicUnit=on
  Out1 : Outport  VectorParamsAs1DForOutWhenUnconnected=off
  wires:
  In1/1 -> Cast To Double/1
  NOT/1(y) -> Cast To Boolean/1
  Cast To Boolean/1 -> Out1/1
  Cast To Double/1 -> NOT/1(u)

== system Control_Logic_e/NOT3 ==
  In1 : Inport
  Cast To Boolean : DataTypeConversion  OutDataTypeStr=boolean
  Cast To Double : DataTypeConversion  OutDataTypeStr=double
  NOT : MATLAB Function  TreatAsAtomicUnit=on
  Out1 : Outport  VectorParamsAs1DForOutWhenUnconnected=off
  wires:
  In1/1 -> Cast To Double/1
  NOT/1(y) -> Cast To Boolean/1
  Cast To Boolean/1 -> Out1/1
  Cast To Double/1 -> NOT/1(u)

== system Control_Logic_e/NOT4 ==
  In1 : Inport
  Cast To Boolean : DataTypeConversion  OutDataTypeStr=boolean
  Cast To Double : DataTypeConversion  OutDataTypeStr=double
  NOT : MATLAB Function  TreatAsAtomicUnit=on
  Out1 : Outport  VectorParamsAs1DForOutWhenUnconnected=off
  wires:
  In1/1 -> Cast To Double/1
  NOT/1(y) -> Cast To Boolean/1
  Cast To Boolean/1 -> Out1/1
  Cast To Double/1 -> NOT/1(u)

== system Control_Logic_e/NOT5 ==
  In1 : Inport
  Cast To Boolean : DataTypeConversion  OutDataTypeStr=boolean
  Cast To Double : DataTypeConversion  OutDataTypeStr=double
  NOT : MATLAB Function  TreatAsAtomicUnit=on
  Out1 : Outport  VectorParamsAs1DForOutWhenUnconnected=off
  wires:
  In1/1 -> Cast To Double/1
  NOT/1(y) -> Cast To Boolean/1
  Cast To Boolean/1 -> Out1/1
  Cast To Double/1 -> NOT/1(u)

== system Control_Logic_e/NOT6 ==
  In1 : Inport
  Cast To Boolean : DataTypeConversion  OutDataTypeStr=boolean
  Cast To Double : DataTypeConversion  OutDataTypeStr=double
  NOT : MATLAB Function  TreatAsAtomicUnit=on
  Out1 : Outport  VectorParamsAs1DForOutWhenUnconnected=off
  wires:
  In1/1 -> Cast To Double/1
  NOT/1(y) -> Cast To Boolean/1
  Cast To Boolean/1 -> Out1/1
  Cast To Double/1 -> NOT/1(u)

== system Control_Logic_e/NOT7 ==
  In1 : Inport
  Cast To Boolean : DataTypeConversion  OutDataTypeStr=boolean
  Cast To Double : DataTypeConversion  OutDataTypeStr=double
  NOT : MATLAB Function  TreatAsAtomicUnit=on
  Out1 : Outport  VectorParamsAs1DForOutWhenUnconnected=off
  wires:
  In1/1 -> Cast To Double/1
  NOT/1(y) -> Cast To Boolean/1
  Cast To Boolean/1 -> Out1/1
  Cast To Double/1 -> NOT/1(u)

== system Control_Logic_e/OFDLC1 ==
  note: y_old
  In : Inport
  Tset : Inport  Port=2
  Cast To Boolean : DataTypeConversion  OutDataTypeStr=boolean
  Cast To Double : DataTypeConversion  OutDataTypeStr=double
  Demux : Demux  Outputs=2
  Memory : Memory  InheritSampleTime=on
  Mux : Mux  Inputs=3
  OFDLC : MATLAB Function  TreatAsAtomicUnit=on
  dt : Constant  Value=Sample_time  OutDataTypeStr=double  SampleTime=Sample_time
  Out : Outport  VectorParamsAs1DForOutWhenUnconnected=off
  wires:
  In/1 -> Cast To Double/1
  Tset/1 -> Mux/2
  Demux/1 -> Cast To Boolean/1
  Demux/2 -> Memory/1
  OFDLC/1(y) -> Demux/1
  Cast To Boolean/1 -> Out/1
  Mux/1 -> OFDLC/1(u)
  dt/1 -> Mux/3
  Cast To Double/1 -> Mux/1
  Memory/1 -> OFDLC/2(old)

== system Control_Logic_e/OFDLC2 ==
  note: y_old
  In : Inport
  Tset : Inport  Port=2
  Cast To Boolean : DataTypeConversion  OutDataTypeStr=boolean
  Cast To Double : DataTypeConversion  OutDataTypeStr=double
  Demux : Demux  Outputs=2
  Memory : Memory  InheritSampleTime=on
  Mux : Mux  Inputs=3
  OFDLC : MATLAB Function  TreatAsAtomicUnit=on
  dt : Constant  Value=Sample_time  OutDataTypeStr=double  SampleTime=Sample_time
  Out : Outport  VectorParamsAs1DForOutWhenUnconnected=off
  wires:
  In/1 -> Cast To Double/1
  Tset/1 -> Mux/2
  Demux/1 -> Cast To Boolean/1
  Demux/2 -> Memory/1
  OFDLC/1(y) -> Demux/1
  Cast To Boolean/1 -> Out/1
  Mux/1 -> OFDLC/1(u)
  dt/1 -> Mux/3
  Cast To Double/1 -> Mux/1
  Memory/1 -> OFDLC/2(old)

== system Control_Logic_e/ONDLC ==
  note: y_old
  In : Inport
  Tset : Inport  Port=2
  Cast To Boolean : DataTypeConversion  OutDataTypeStr=boolean
  Cast To Double : DataTypeConversion  OutDataTypeStr=double
  Demux : Demux  Outputs=2
  Memory : Memory  InheritSampleTime=on
  Mux : Mux  Inputs=3
  ONDLC : MATLAB Function  TreatAsAtomicUnit=on
  dt : Constant  Value=Sample_time  OutDataTypeStr=double  SampleTime=Sample_time
  Out : Outport  VectorParamsAs1DForOutWhenUnconnected=off
  wires:
  In/1 -> Cast To Double/1
  Tset/1 -> Mux/2
  Demux/1 -> Cast To Boolean/1
  Demux/2 -> Memory/1
  ONDLC/1(y) -> Demux/1
  Cast To Boolean/1 -> Out/1
  Mux/1 -> ONDLC/1(u)
  dt/1 -> Mux/3
  Cast To Double/1 -> Mux/1
  Memory/1 -> ONDLC/2(old)

== system Control_Logic_e/ONDLC1 ==
  note: y_old
  In : Inport
  Tset : Inport  Port=2
  Cast To Boolean : DataTypeConversion  OutDataTypeStr=boolean
  Cast To Double : DataTypeConversion  OutDataTypeStr=double
  Demux : Demux  Outputs=2
  Memory : Memory  InheritSampleTime=on
  Mux : Mux  Inputs=3
  ONDLC : MATLAB Function  TreatAsAtomicUnit=on
  dt : Constant  Value=Sample_time  OutDataTypeStr=double  SampleTime=Sample_time
  Out : Outport  VectorParamsAs1DForOutWhenUnconnected=off
  wires:
  In/1 -> Cast To Double/1
  Tset/1 -> Mux/2
  Demux/1 -> Cast To Boolean/1
  Demux/2 -> Memory/1
  ONDLC/1(y) -> Demux/1
  Cast To Boolean/1 -> Out/1
  Mux/1 -> ONDLC/1(u)
  dt/1 -> Mux/3
  Cast To Double/1 -> Mux/1
  Memory/1 -> ONDLC/2(old)

== system Control_Logic_e/ONDLC2 ==
  note: y_old
  In : Inport
  Tset : Inport  Port=2
  Cast To Boolean : DataTypeConversion  OutDataTypeStr=boolean
  Cast To Double : DataTypeConversion  OutDataTypeStr=double
  Demux : Demux  Outputs=2
  Memory : Memory  InheritSampleTime=on
  Mux : Mux  Inputs=3
  ONDLC : MATLAB Function  TreatAsAtomicUnit=on
  dt : Constant  Value=Sample_time  OutDataTypeStr=double  SampleTime=Sample_time
  Out : Outport  VectorParamsAs1DForOutWhenUnconnected=off
  wires:
  In/1 -> Cast To Double/1
  Tset/1 -> Mux/2
  Demux/1 -> Cast To Boolean/1
  Demux/2 -> Memory/1
  ONDLC/1(y) -> Demux/1
  Cast To Boolean/1 -> Out/1
  Mux/1 -> ONDLC/1(u)
  dt/1 -> Mux/3
  Cast To Double/1 -> Mux/1
  Memory/1 -> ONDLC/2(old)

== system Control_Logic_e/ONDLC3 ==
  note: y_old
  In : Inport
  Tset : Inport  Port=2
  Cast To Boolean : DataTypeConversion  OutDataTypeStr=boolean
  Cast To Double : DataTypeConversion  OutDataTypeStr=double
  Demux : Demux  Outputs=2
  Memory : Memory  InheritSampleTime=on
  Mux : Mux  Inputs=3
  ONDLC : MATLAB Function  TreatAsAtomicUnit=on
  dt : Constant  Value=Sample_time  OutDataTypeStr=double  SampleTime=Sample_time
  Out : Outport  VectorParamsAs1DForOutWhenUnconnected=off
  wires:
  In/1 -> Cast To Double/1
  Tset/1 -> Mux/2
  Demux/1 -> Cast To Boolean/1
  Demux/2 -> Memory/1
  ONDLC/1(y) -> Demux/1
  Cast To Boolean/1 -> Out/1
  Mux/1 -> ONDLC/1(u)
  dt/1 -> Mux/3
  Cast To Double/1 -> Mux/1
  Memory/1 -> ONDLC/2(old)

== system Control_Logic_e/ONDLC6 ==
  note: y_old
  In : Inport
  Tset : Inport  Port=2
  Cast To Boolean : DataTypeConversion  OutDataTypeStr=boolean
  Cast To Double : DataTypeConversion  OutDataTypeStr=double
  Demux : Demux  Outputs=2
  Memory : Memory  InheritSampleTime=on
  Mux : Mux  Inputs=3
  ONDLC : MATLAB Function  TreatAsAtomicUnit=on
  dt : Constant  Value=Sample_time  OutDataTypeStr=double  SampleTime=Sample_time
  Out : Outport  VectorParamsAs1DForOutWhenUnconnected=off
  wires:
  Memory/1 -> ONDLC/2(old)
  Cast To Double/1 -> Mux/1
  dt/1 -> Mux/3
  Mux/1 -> ONDLC/1(u)
  Cast To Boolean/1 -> Out/1
  ONDLC/1(y) -> Demux/1
  Demux/2 -> Memory/1
  Demux/1 -> Cast To Boolean/1
  Tset/1 -> Mux/2
  In/1 -> Cast To Double/1

== system Control_Logic_e/ONDLC7 ==
  note: y_old
  In : Inport
  Tset : Inport  Port=2
  Cast To Boolean : DataTypeConversion  OutDataTypeStr=boolean
  Cast To Double : DataTypeConversion  OutDataTypeStr=double
  Demux : Demux  Outputs=2
  Memory : Memory  InheritSampleTime=on
  Mux : Mux  Inputs=3
  ONDLC : MATLAB Function  TreatAsAtomicUnit=on
  dt : Constant  Value=Sample_time  OutDataTypeStr=double  SampleTime=Sample_time
  Out : Outport  VectorParamsAs1DForOutWhenUnconnected=off
  wires:
  In/1 -> Cast To Double/1
  Tset/1 -> Mux/2
  Demux/1 -> Cast To Boolean/1
  Demux/2 -> Memory/1
  ONDLC/1(y) -> Demux/1
  Cast To Boolean/1 -> Out/1
  Mux/1 -> ONDLC/1(u)
  dt/1 -> Mux/3
  Cast To Double/1 -> Mux/1
  Memory/1 -> ONDLC/2(old)

== system Control_Logic_e/OR ==
  In1 : Inport
  In2 : Inport  Port=2
  Cast To Boolean : DataTypeConversion  OutDataTypeStr=boolean
  Cast To Double : DataTypeConversion  OutDataTypeStr=double
  MATLAB Function : MATLAB Function  TreatAsAtomicUnit=on
  Mux : Mux  Inputs=2
  Out : Outport  VectorParamsAs1DForOutWhenUnconnected=off
  wires:
  Mux/1 -> Cast To Double/1
  MATLAB Function/1(y) -> Cast To Boolean/1
  In1/1 -> Mux/1
  In2/1 -> Mux/2
  Cast To Double/1 -> MATLAB Function/1(u)
  Cast To Boolean/1 -> Out/1

== system Control_Logic_e/OR1 ==
  In1 : Inport
  In2 : Inport  Port=2
  Cast To Boolean : DataTypeConversion  OutDataTypeStr=boolean
  Cast To Double : DataTypeConversion  OutDataTypeStr=double
  MATLAB Function : MATLAB Function  TreatAsAtomicUnit=on
  Mux : Mux  Inputs=2
  Out : Outport  VectorParamsAs1DForOutWhenUnconnected=off
  wires:
  Mux/1 -> Cast To Double/1
  MATLAB Function/1(y) -> Cast To Boolean/1
  In1/1 -> Mux/1
  In2/1 -> Mux/2
  Cast To Double/1 -> MATLAB Function/1(u)
  Cast To Boolean/1 -> Out/1

== system Control_Logic_e/OR2 ==
  In1 : Inport
  In2 : Inport  Port=2
  Cast To Boolean : DataTypeConversion  OutDataTypeStr=boolean
  Cast To Double : DataTypeConversion  OutDataTypeStr=double
  MATLAB Function : MATLAB Function  TreatAsAtomicUnit=on
  Mux : Mux  Inputs=2
  Out : Outport  VectorParamsAs1DForOutWhenUnconnected=off
  wires:
  Mux/1 -> Cast To Double/1
  MATLAB Function/1(y) -> Cast To Boolean/1
  In1/1 -> Mux/1
  In2/1 -> Mux/2
  Cast To Double/1 -> MATLAB Function/1(u)
  Cast To Boolean/1 -> Out/1

== system Control_Logic_e/OR3 ==
  In1 : Inport
  In2 : Inport  Port=2
  In3 : Inport  Port=3
  Cast To Boolean : DataTypeConversion  OutDataTypeStr=boolean
  Cast To Double : DataTypeConversion  OutDataTypeStr=double
  Cast To Double1 : DataTypeConversion  OutDataTypeStr=double
  Cast To Double2 : DataTypeConversion  OutDataTypeStr=double
  MATLAB Function : MATLAB Function  TreatAsAtomicUnit=on
  Mux : Mux  Inputs=3
  Out : Outport  VectorParamsAs1DForOutWhenUnconnected=off
  wires:
  MATLAB Function/1(y) -> Cast To Boolean/1
  Mux/1 -> MATLAB Function/1(u)
  Cast To Boolean/1 -> Out/1
  In1/1 -> Cast To Double/1
  In2/1 -> Cast To Double1/1
  In3/1 -> Cast To Double2/1
  Cast To Double/1 -> Mux/1
  Cast To Double1/1 -> Mux/2
  Cast To Double2/1 -> Mux/3

== system Control_Logic_e/OR4 ==
  In1 : Inport
  In2 : Inport  Port=2
  In3 : Inport  Port=3
  Cast To Boolean : DataTypeConversion  OutDataTypeStr=boolean
  Cast To Double : DataTypeConversion  OutDataTypeStr=double
  Cast To Double1 : DataTypeConversion  OutDataTypeStr=double
  Cast To Double2 : DataTypeConversion  OutDataTypeStr=double
  MATLAB Function : MATLAB Function  TreatAsAtomicUnit=on
  Mux : Mux  Inputs=3
  Out : Outport  VectorParamsAs1DForOutWhenUnconnected=off
  wires:
  MATLAB Function/1(y) -> Cast To Boolean/1
  Mux/1 -> MATLAB Function/1(u)
  Cast To Boolean/1 -> Out/1
  In1/1 -> Cast To Double/1
  In2/1 -> Cast To Double1/1
  In3/1 -> Cast To Double2/1
  Cast To Double/1 -> Mux/1
  Cast To Double1/1 -> Mux/2
  Cast To Double2/1 -> Mux/3

== system Control_Logic_e/OR5 ==
  In1 : Inport
  In2 : Inport  Port=2
  In3 : Inport  Port=3
  Cast To Boolean : DataTypeConversion  OutDataTypeStr=boolean
  Cast To Double : DataTypeConversion  OutDataTypeStr=double
  Cast To Double1 : DataTypeConversion  OutDataTypeStr=double
  Cast To Double2 : DataTypeConversion  OutDataTypeStr=double
  MATLAB Function : MATLAB Function  TreatAsAtomicUnit=on
  Mux : Mux  Inputs=3
  Out : Outport  VectorParamsAs1DForOutWhenUnconnected=off
  wires:
  MATLAB Function/1(y) -> Cast To Boolean/1
  Cast To Boolean/1 -> Out/1
  Mux/1 -> MATLAB Function/1(u)
  In1/1 -> Cast To Double/1
  In2/1 -> Cast To Double1/1
  In3/1 -> Cast To Double2/1
  Cast To Double/1 -> Mux/1
  Cast To Double1/1 -> Mux/2
  Cast To Double2/1 -> Mux/3

== system Control_Logic_e/OR6 ==
  In1 : Inport
  In2 : Inport  Port=2
  In3 : Inport  Port=3
  Cast To Boolean : DataTypeConversion  OutDataTypeStr=boolean
  Cast To Double : DataTypeConversion  OutDataTypeStr=double
  Cast To Double1 : DataTypeConversion  OutDataTypeStr=double
  Cast To Double2 : DataTypeConversion  OutDataTypeStr=double
  MATLAB Function : MATLAB Function  TreatAsAtomicUnit=on
  Mux : Mux  Inputs=3
  Out : Outport  VectorParamsAs1DForOutWhenUnconnected=off
  wires:
  MATLAB Function/1(y) -> Cast To Boolean/1
  Cast To Boolean/1 -> Out/1
  Mux/1 -> MATLAB Function/1(u)
  In1/1 -> Cast To Double/1
  In2/1 -> Cast To Double1/1
  In3/1 -> Cast To Double2/1
  Cast To Double/1 -> Mux/1
  Cast To Double1/1 -> Mux/2
  Cast To Double2/1 -> Mux/3

== system Control_Logic_e/OR7 ==
  In1 : Inport
  In2 : Inport  Port=2
  Cast To Boolean : DataTypeConversion  OutDataTypeStr=boolean
  Cast To Double : DataTypeConversion  OutDataTypeStr=double
  MATLAB Function : MATLAB Function  TreatAsAtomicUnit=on
  Mux : Mux  Inputs=2
  Out : Outport  VectorParamsAs1DForOutWhenUnconnected=off
  wires:
  Mux/1 -> Cast To Double/1
  MATLAB Function/1(y) -> Cast To Boolean/1
  In1/1 -> Mux/1
  In2/1 -> Mux/2
  Cast To Double/1 -> MATLAB Function/1(u)
  Cast To Boolean/1 -> Out/1

== system Control_Logic_e/OR8 ==
  In1 : Inport
  In2 : Inport  Port=2
  In3 : Inport  Port=3
  Cast To Boolean : DataTypeConversion  OutDataTypeStr=boolean
  Cast To Double : DataTypeConversion  OutDataTypeStr=double
  Cast To Double1 : DataTypeConversion  OutDataTypeStr=double
  Cast To Double2 : DataTypeConversion  OutDataTypeStr=double
  MATLAB Function : MATLAB Function  TreatAsAtomicUnit=on
  Mux : Mux  Inputs=3
  Out : Outport  VectorParamsAs1DForOutWhenUnconnected=off
  wires:
  MATLAB Function/1(y) -> Cast To Boolean/1
  Cast To Boolean/1 -> Out/1
  Mux/1 -> MATLAB Function/1(u)
  In1/1 -> Cast To Double/1
  In2/1 -> Cast To Double1/1
  In3/1 -> Cast To Double2/1
  Cast To Double/1 -> Mux/1
  Cast To Double1/1 -> Mux/2
  Cast To Double2/1 -> Mux/3

== system Control_Logic_e/OR9 ==
  In1 : Inport
  In2 : Inport  Port=2
  In3 : Inport  Port=3
  Cast To Boolean : DataTypeConversion  OutDataTypeStr=boolean
  Cast To Double : DataTypeConversion  OutDataTypeStr=double
  Cast To Double1 : DataTypeConversion  OutDataTypeStr=double
  Cast To Double2 : DataTypeConversion  OutDataTypeStr=double
  MATLAB Function : MATLAB Function  TreatAsAtomicUnit=on
  Mux : Mux  Inputs=3
  Out : Outport  VectorParamsAs1DForOutWhenUnconnected=off
  wires:
  MATLAB Function/1(y) -> Cast To Boolean/1
  Cast To Boolean/1 -> Out/1
  Mux/1 -> MATLAB Function/1(u)
  In1/1 -> Cast To Double/1
  In2/1 -> Cast To Double1/1
  In3/1 -> Cast To Double2/1
  Cast To Double/1 -> Mux/1
  Cast To Double1/1 -> Mux/2
  Cast To Double2/1 -> Mux/3

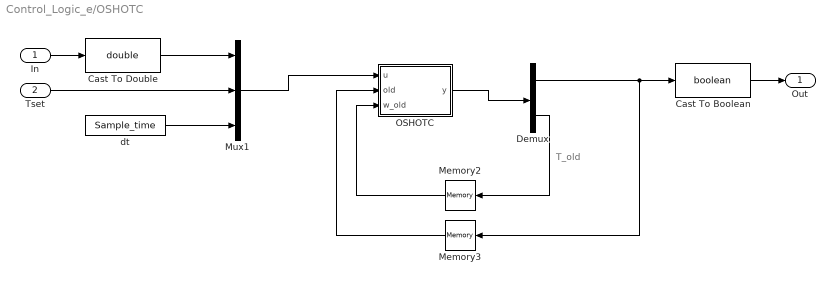
== system Control_Logic_e/OSHOTC ==
  note: T_old
  In : Inport
  Tset : Inport  Port=2
  Cast To Boolean : DataTypeConversion  OutDataTypeStr=boolean
  Cast To Double : DataTypeConversion  OutDataTypeStr=double
  Demux : Demux  Outputs=2
  Memory2 : Memory  InheritSampleTime=on
  Memory3 : Memory  InheritSampleTime=on  LinearizeAsDelay=on
  Mux1 : Mux  Inputs=3
  OSHOTC : MATLAB Function  TreatAsAtomicUnit=on
  dt : Constant  Value=Sample_time  OutDataTypeStr=double  SampleTime=Sample_time
  Out : Outport  VectorParamsAs1DForOutWhenUnconnected=off
  wires:
  OSHOTC/1(y) -> Demux/1
  Demux/1 -> Memory3/1, Cast To Boolean/1
  Cast To Boolean/1 -> Out/1
  Mux1/1 -> OSHOTC/1(u)
  Demux/2 -> Memory2/1
  Memory2/1 -> OSHOTC/3(w_old)
  dt/1 -> Mux1/3
  Tset/1 -> Mux1/2
  Memory3/1 -> OSHOTC/2(old)
  In/1 -> Cast To Double/1
  Cast To Double/1 -> Mux1/1
